simulink model "SIMULINK_PID_Tracking_R18b"  (R2018b)
settings: Solver=FixedStepAuto  StartTime=0.0  StopTime=sim_end_time  FixedStep=fixed_step_size  RelTol=1e-3
undefined symbols (not defined in the file): a, act_end, b, battery_threshold, bb, draw_gif, droneyeeUAV2_NUM, droneyeeUAV3_NUM, droneyeeUAV4_NUM, droneyeeUAV5_NUM, fixed_step_size, k, KD_x, KD_y, kd_z, KDD_x, KDD_y, KI_x, KI_y, ki_z, KII_x, KII_y, KP_x, KP_y, kp_z, KPP_x, KPP_y, lmt, omega, R, sim_end_time, uav10num, uav1num, uav2num, uav3num, uav4num, uav5num, uav6num, uav7num, uav8num, uav9num, UAV_NUM, Vel_Switch_1, Vel_Switch_10, Vel_Switch_11, Vel_Switch_12, Vel_Switch_13, Vel_Switch_14, Vel_Switch_15, Vel_Switch_16, Vel_Switch_17, Vel_Switch_18, Vel_Switch_19, Vel_Switch_2, Vel_Switch_20, Vel_Switch_3, Vel_Switch_4, Vel_Switch_5, Vel_Switch_6, Vel_Switch_7 ... (+12)
libraries: simulink x120, aerolibanimutils x1
(part 10 of 10)

== matlab function SIMULINK_PID_Tracking_R18b/防碰撞2/MATLAB Function ==
  settings: updateMethod=DISCRETE
  data: u1 input; xd output; u2 input; yd output; zd output; u3 input; u4 input; u5 input; flag input
function [xd,yd,zd] = fcn(u1,u2,u3,u4,u5,flag)
persistent xdd ydd zdd xtt ytt ztt;
k=u4;
totnum =10;
safedist =u3;%安全距离的平方
bang=u5;
xdd=zeros(totnum,1);
ydd=zeros(totnum,1);
zdd=zeros(totnum,1);
xt=zeros(totnum,1);
yt=zeros(totnum,1);
zt=zeros(totnum,1);
vx=xt;
vy=yt;
vz=zt;
xd=xt;
yd=yt;
zd=zt;
for i =1:1:totnum
    xt(i)=u2(12*(i-1)+1);
    yt(i)=u2(12*(i-1)+2);
    zt(i)=u2(12*(i-1)+3);
    xd(i)=u1(6*(i-1)+1);
    yd(i)=u1(6*(i-1)+2);
    zd(i)=u1(6*(i-1)+3);
    vx(i)=u2(12*(i-1)+10);
    vy(i)=u2(12*(i-1)+11);
    vz(i)=u2(12*(i-1)+12);
end
if flag==1
if isempty(xt)
    xtt = xt;
    ytt = yt;
    ztt = zt;
end
for i =1:1:(totnum-1)
    if xt(i)==0&&yt(i)==0&&zt(i)==0
        break
    end
    for j=(i+1):1:totnum
        if xt(j)==0&&yt(j)==0&&zt(j)==0
        break
        end
        dist=((xt(i)-xt(j))^2+(yt(i)-yt(j))^2+(zt(i)-zt(j))^2);
        sqrt_dist=sqrt((xt(i)-xt(j))^2+(yt(i)-yt(j))^2);
    if (dist>0)&&(sqrt(dist)<=bang)
%         xd(i)=xt(i);
%         yd(i)=yt(i);
%         zd(i)=0; %zt(i);
%         xd(j)=xt(j);
%         yd(j)=yt(j);
%         zd(j)=zt(j);        
%         xd(i)=xd(i)+k*(xt(i)-xt(j))*(safedist-dist);
%         yd(i)=yd(i)+k*(yt(i)-yt(j))*(safedist-dist);
        xdd(i)=xdd(i)+k*(xt(i)-xt(j))*(safedist-dist);
        ydd(i)=ydd(i)+k*(yt(i)-yt(j))*(safedist-dist);
%         zd(i)=zd(i)+k*(zt(i)-zt(j))*(safedist-dist);
%         xd(j)=xd(j)-k*(xt(i)-xt(j))*(safedist-dist);
%         yd(j)=yd(j)-k*(yt(i)-yt(j))*(safedist-dist);
        xdd(j)=xdd(j)-k*(xt(i)-xt(j))*(safedist-dist);
        ydd(j)=ydd(j)-k*(yt(i)-yt(j))*(safedist-dist);
%         zd(j)=zd(j)-k*(zt(i)-zt(j))*(safedist-dist);
     elseif (sqrt(dist)<safedist)&&(((vx(i)-vx(j))*(xt(i)-xt(j))+...
             (vy(i)-vy(j))*(yt(i)-yt(j)))<0)
%         dist=dist-bang;
%         xd(i)=xd(i)+k*(yt(i)-yt(j))*(safedist-dist);
%         yd(i)=yd(i)+k*(xt(j)-xt(i))*(safedist-dist);
        xdd(i)=xdd(i)+k*(yt(i)-yt(j))*(safedist-sqrt_dist)/sqrt_dist/sqrt_dist;
        ydd(i)=ydd(i)+k*(xt(j)-xt(i))*(safedist-sqrt_dist)/sqrt_dist/sqrt_dist;
%         zd(i)=zd(i)+k*(zt(i)-zt(j))*(safedist-dist);
%         xd(j)=xd(j)-k*(yt(i)-yt(j))*(safedist-dist);
%         yd(j)=yd(j)-k*(xt(j)-xt(i))*(safedist-dist);
        xdd(j)=xdd(j)-k*(yt(i)-yt(j))*(safedist-sqrt_dist)/sqrt_dist/sqrt_dist;
        ydd(j)=ydd(j)-k*(xt(j)-xt(i))*(safedist-sqrt_dist)/sqrt_dist/sqrt_dist;
%         zd(j)=zd(j)-k*(zt(i)-zt(j))*(safedist-dist);
        
    end
    end
end
xd=xd+xdd;
yd=yd+ydd;
% zd=zdd;
end

== matlab function SIMULINK_PID_Tracking_R18b/control system_UAV/Baseline Controller3/MATLAB Function ==
  data: u input; y output; a input
function y = fcn(u,a)
y = satgd(u,a);

== matlab function SIMULINK_PID_Tracking_R18b/CMD_car1/CMD6/Subsystem/MATLAB Function ==
  settings: updateMethod=DISCRETE
  data: timestamp input; uavnum input; x_ output; y_ output; z_ output; switch_flag input; stas input; trj_flag input; form_flag input; avo_flag input
function [x_, y_, z_] = fcn(timestamp, uavnum,switch_flag,stas,trj_flag,form_flag,avo_flag)

[x_,y_,z_]=trjcar(timestamp,uavnum,switch_flag,stas,trj_flag,form_flag,avo_flag);

== matlab function SIMULINK_PID_Tracking_R18b/control system_UAV/Baseline Controller4/MATLAB Function ==
  data: u input; y output; a input
function y = fcn(u,a)
y = satgd(u,a);

== matlab function SIMULINK_PID_Tracking_R18b/CMD_car1/CMD7/MATLAB Function1 ==
  settings: updateMethod=DISCRETE
  data: x_d input; y_d input; z_d input; timestamp input; x input; y input; z input; battery_status input; sim_time_end input; x_d_ output; battery_threshold input; z_d_for_land input; y_d_ output; z_d_ output; UAV_NUM input
function [x_d_, y_d_, z_d_] = fcn(x_d, y_d, z_d, timestamp, x,y,z,battery_status, sim_time_end,battery_threshold, z_d_for_land, UAV_NUM)
persistent s_x s_y s_z ready_land
if isempty(s_x)
    s_x = x;
end
if isempty(s_y)
    s_y = y;
end
if isempty(s_z)
    s_z = z;
end
if isempty(ready_land)
    ready_land = false;
end
    
battery_low = false;
for i = 1:UAV_NUM
    if battery_status(i) < battery_threshold
        battery_low = true;
        break;
    end
end
if sim_time_end - timestamp < 1
    tello_stop = true;
else
    tello_stop = false;
end
if battery_low || tello_stop
    if ~ready_land
        ready_land = true;
    end
    z_d_ = z_d_for_land;
    x_d_ = s_x;
    y_d_ = s_y;
else
   ready_land = false;
   s_x = x;
   s_y = y;
   x_d_ = x_d;
   y_d_ = y_d;
   z_d_ = z_d;
end

== matlab function SIMULINK_PID_Tracking_R18b/CMD_UAV/CMD6/Subsystem/MATLAB Function ==
  settings: updateMethod=DISCRETE
  data: timestamp input; uavnum input; x_ output; y_ output; z_ output; switch_flag input; stas input; trj_flag input; form_flag input; avo_flag input
function [x_, y_, z_] = fcn(timestamp, uavnum,switch_flag,stas,trj_flag,form_flag,avo_flag)

[x_,y_,z_]=trjuav(timestamp,uavnum,switch_flag,stas,trj_flag,form_flag,avo_flag);

== matlab function SIMULINK_PID_Tracking_R18b/CMD_UAV/CMD7/MATLAB Function1 ==
  settings: updateMethod=DISCRETE
  data: x_d input; y_d input; z_d input; timestamp input; x input; y input; z input; battery_status input; sim_time_end input; x_d_ output; battery_threshold input; z_d_for_land input; y_d_ output; z_d_ output; UAV_NUM input
function [x_d_, y_d_, z_d_] = fcn(x_d, y_d, z_d, timestamp, x,y,z,battery_status, sim_time_end,battery_threshold, z_d_for_land, UAV_NUM)
persistent s_x s_y s_z ready_land
if isempty(s_x)
    s_x = x;
end
if isempty(s_y)
    s_y = y;
end
if isempty(s_z)
    s_z = z;
end
if isempty(ready_land)
    ready_land = false;
end
    
battery_low = false;
for i = 1:UAV_NUM
    if battery_status(i) < battery_threshold
        battery_low = true;
        break;
    end
end
if sim_time_end - timestamp < 1
    tello_stop = true;
else
    tello_stop = false;
end
if battery_low || tello_stop
    if ~ready_land
        ready_land = true;
    end
    z_d_ = z_d_for_land;
    x_d_ = s_x;
    y_d_ = s_y;
else
   ready_land = false;
   s_x = x;
   s_y = y;
   x_d_ = x_d;
   y_d_ = y_d;
   z_d_ = z_d;
end

== matlab function SIMULINK_PID_Tracking_R18b/CMD_UAV/CMD7/Subsystem/MATLAB Function ==
  settings: updateMethod=DISCRETE
  data: timestamp input; uavnum input; x_ output; y_ output; z_ output; switch_flag input; stas input; trj_flag input; form_flag input; avo_flag input
function [x_, y_, z_] = fcn(timestamp, uavnum,switch_flag,stas,trj_flag,form_flag,avo_flag)

[x_,y_,z_]=trjuav(timestamp,uavnum,switch_flag,stas,trj_flag,form_flag,avo_flag);

== matlab function SIMULINK_PID_Tracking_R18b/CMD_UAV/CMD8/MATLAB Function1 ==
  settings: updateMethod=DISCRETE
  data: x_d input; y_d input; z_d input; timestamp input; x input; y input; z input; battery_status input; sim_time_end input; x_d_ output; battery_threshold input; z_d_for_land input; y_d_ output; z_d_ output; UAV_NUM input
function [x_d_, y_d_, z_d_] = fcn(x_d, y_d, z_d, timestamp, x,y,z,battery_status, sim_time_end,battery_threshold, z_d_for_land, UAV_NUM)
persistent s_x s_y s_z ready_land
if isempty(s_x)
    s_x = x;
end
if isempty(s_y)
    s_y = y;
end
if isempty(s_z)
    s_z = z;
end
if isempty(ready_land)
    ready_land = false;
end
    
battery_low = false;
for i = 1:UAV_NUM
    if battery_status(i) < battery_threshold
        battery_low = true;
        break;
    end
end
if sim_time_end - timestamp < 1
    tello_stop = true;
else
    tello_stop = false;
end
if battery_low || tello_stop
    if ~ready_land
        ready_land = true;
    end
    z_d_ = z_d_for_land;
    x_d_ = s_x;
    y_d_ = s_y;
else
   ready_land = false;
   s_x = x;
   s_y = y;
   x_d_ = x_d;
   y_d_ = y_d;
   z_d_ = z_d;
end

== matlab function SIMULINK_PID_Tracking_R18b/CMD_UAV/CMD8/Subsystem/MATLAB Function ==
  settings: updateMethod=DISCRETE
  data: timestamp input; uavnum input; x_ output; y_ output; z_ output; switch_flag input; stas input; trj_flag input; form_flag input; avo_flag input
function [x_, y_, z_] = fcn(timestamp, uavnum,switch_flag,stas,trj_flag,form_flag,avo_flag)

[x_,y_,z_]=trjuav(timestamp,uavnum,switch_flag,stas,trj_flag,form_flag,avo_flag);

== matlab function SIMULINK_PID_Tracking_R18b/CMD_UAV/CMD10/MATLAB Function1 ==
  settings: updateMethod=DISCRETE
  data: x_d input; y_d input; z_d input; timestamp input; x input; y input; z input; battery_status input; sim_time_end input; x_d_ output; battery_threshold input; z_d_for_land input; y_d_ output; z_d_ output; UAV_NUM input
function [x_d_, y_d_, z_d_] = fcn(x_d, y_d, z_d, timestamp, x,y,z,battery_status, sim_time_end,battery_threshold, z_d_for_land, UAV_NUM)
persistent s_x s_y s_z ready_land
if isempty(s_x)
    s_x = x;
end
if isempty(s_y)
    s_y = y;
end
if isempty(s_z)
    s_z = z;
end
if isempty(ready_land)
    ready_land = false;
end
    
battery_low = false;
for i = 1:UAV_NUM
    if battery_status(i) < battery_threshold
        battery_low = true;
        break;
    end
end
if sim_time_end - timestamp < 1
    tello_stop = true;
else
    tello_stop = false;
end
if battery_low || tello_stop
    if ~ready_land
        ready_land = true;
    end
    z_d_ = z_d_for_land;
    x_d_ = s_x;
    y_d_ = s_y;
else
   ready_land = false;
   s_x = x;
   s_y = y;
   x_d_ = x_d;
   y_d_ = y_d;
   z_d_ = z_d;
end

== matlab function SIMULINK_PID_Tracking_R18b/CMD_UAV/CMD10/Subsystem/MATLAB Function ==
  settings: updateMethod=DISCRETE
  data: timestamp input; uavnum input; x_ output; y_ output; z_ output; switch_flag input; stas input; trj_flag input; form_flag input; avo_flag input
function [x_, y_, z_] = fcn(timestamp, uavnum,switch_flag,stas,trj_flag,form_flag,avo_flag)

[x_,y_,z_]=trjuav(timestamp,uavnum,switch_flag,stas,trj_flag,form_flag,avo_flag);

== matlab function SIMULINK_PID_Tracking_R18b/CMD_UAV/CMD9/MATLAB Function1 ==
  settings: updateMethod=DISCRETE
  data: x_d input; y_d input; z_d input; timestamp input; x input; y input; z input; battery_status input; sim_time_end input; x_d_ output; battery_threshold input; z_d_for_land input; y_d_ output; z_d_ output; UAV_NUM input
function [x_d_, y_d_, z_d_] = fcn(x_d, y_d, z_d, timestamp, x,y,z,battery_status, sim_time_end,battery_threshold, z_d_for_land, UAV_NUM)
persistent s_x s_y s_z ready_land
if isempty(s_x)
    s_x = x;
end
if isempty(s_y)
    s_y = y;
end
if isempty(s_z)
    s_z = z;
end
if isempty(ready_land)
    ready_land = false;
end
    
battery_low = false;
for i = 1:UAV_NUM
    if battery_status(i) < battery_threshold
        battery_low = true;
        break;
    end
end
if sim_time_end - timestamp < 1
    tello_stop = true;
else
    tello_stop = false;
end
if battery_low || tello_stop
    if ~ready_land
        ready_land = true;
    end
    z_d_ = z_d_for_land;
    x_d_ = s_x;
    y_d_ = s_y;
else
   ready_land = false;
   s_x = x;
   s_y = y;
   x_d_ = x_d;
   y_d_ = y_d;
   z_d_ = z_d;
end

== matlab function SIMULINK_PID_Tracking_R18b/CMD_UAV/CMD9/Subsystem/MATLAB Function ==
  settings: updateMethod=DISCRETE
  data: timestamp input; uavnum input; x_ output; y_ output; z_ output; switch_flag input; stas input; trj_flag input; form_flag input; avo_flag input
function [x_, y_, z_] = fcn(timestamp, uavnum,switch_flag,stas,trj_flag,form_flag,avo_flag)

[x_,y_,z_]=trjuav(timestamp,uavnum,switch_flag,stas,trj_flag,form_flag,avo_flag);

== matlab function SIMULINK_PID_Tracking_R18b/CMD_car1/CMD7/Subsystem/MATLAB Function ==
  settings: updateMethod=DISCRETE
  data: timestamp input; uavnum input; x_ output; y_ output; z_ output; switch_flag input; stas input; trj_flag input; form_flag input; avo_flag input
function [x_, y_, z_] = fcn(timestamp, uavnum,switch_flag,stas,trj_flag,form_flag,avo_flag)

[x_,y_,z_]=trjcar(timestamp,uavnum,switch_flag,stas,trj_flag,form_flag,avo_flag);

== matlab function SIMULINK_PID_Tracking_R18b/CMD_car1/CMD8/MATLAB Function1 ==
  settings: updateMethod=DISCRETE
  data: x_d input; y_d input; z_d input; timestamp input; x input; y input; z input; battery_status input; sim_time_end input; x_d_ output; battery_threshold input; z_d_for_land input; y_d_ output; z_d_ output; UAV_NUM input
function [x_d_, y_d_, z_d_] = fcn(x_d, y_d, z_d, timestamp, x,y,z,battery_status, sim_time_end,battery_threshold, z_d_for_land, UAV_NUM)
persistent s_x s_y s_z ready_land
if isempty(s_x)
    s_x = x;
end
if isempty(s_y)
    s_y = y;
end
if isempty(s_z)
    s_z = z;
end
if isempty(ready_land)
    ready_land = false;
end
    
battery_low = false;
for i = 1:UAV_NUM
    if battery_status(i) < battery_threshold
        battery_low = true;
        break;
    end
end
if sim_time_end - timestamp < 1
    tello_stop = true;
else
    tello_stop = false;
end
if battery_low || tello_stop
    if ~ready_land
        ready_land = true;
    end
    z_d_ = z_d_for_land;
    x_d_ = s_x;
    y_d_ = s_y;
else
   ready_land = false;
   s_x = x;
   s_y = y;
   x_d_ = x_d;
   y_d_ = y_d;
   z_d_ = z_d;
end

== matlab function SIMULINK_PID_Tracking_R18b/CMD_car1/CMD8/Subsystem/MATLAB Function ==
  settings: updateMethod=DISCRETE
  data: timestamp input; uavnum input; x_ output; y_ output; z_ output; switch_flag input; stas input; trj_flag input; form_flag input; avo_flag input
function [x_, y_, z_] = fcn(timestamp, uavnum,switch_flag,stas,trj_flag,form_flag,avo_flag)

[x_,y_,z_]=trjcar(timestamp,uavnum,switch_flag,stas,trj_flag,form_flag,avo_flag);

== matlab function SIMULINK_PID_Tracking_R18b/CMD_car1/CMD9/MATLAB Function1 ==
  settings: updateMethod=DISCRETE
  data: x_d input; y_d input; z_d input; timestamp input; x input; y input; z input; battery_status input; sim_time_end input; x_d_ output; battery_threshold input; z_d_for_land input; y_d_ output; z_d_ output; UAV_NUM input
function [x_d_, y_d_, z_d_] = fcn(x_d, y_d, z_d, timestamp, x,y,z,battery_status, sim_time_end,battery_threshold, z_d_for_land, UAV_NUM)
persistent s_x s_y s_z ready_land
if isempty(s_x)
    s_x = x;
end
if isempty(s_y)
    s_y = y;
end
if isempty(s_z)
    s_z = z;
end
if isempty(ready_land)
    ready_land = false;
end
    
battery_low = false;
for i = 1:UAV_NUM
    if battery_status(i) < battery_threshold
        battery_low = true;
        break;
    end
end
if sim_time_end - timestamp < 1
    tello_stop = true;
else
    tello_stop = false;
end
if battery_low || tello_stop
    if ~ready_land
        ready_land = true;
    end
    z_d_ = z_d_for_land;
    x_d_ = s_x;
    y_d_ = s_y;
else
   ready_land = false;
   s_x = x;
   s_y = y;
   x_d_ = x_d;
   y_d_ = y_d;
   z_d_ = z_d;
end

== matlab function SIMULINK_PID_Tracking_R18b/CMD_car1/CMD9/Subsystem/MATLAB Function ==
  settings: updateMethod=DISCRETE
  data: timestamp input; uavnum input; x_ output; y_ output; z_ output; switch_flag input; stas input; trj_flag input; form_flag input; avo_flag input
function [x_, y_, z_] = fcn(timestamp, uavnum,switch_flag,stas,trj_flag,form_flag,avo_flag)

[x_,y_,z_]=trjcar(timestamp,uavnum,switch_flag,stas,trj_flag,form_flag,avo_flag);

== matlab function SIMULINK_PID_Tracking_R18b/control system_car1/Baseline Controller1/MATLAB Function ==
  data: u input; y output; a input
function y = fcn(u,a)
y = satgd(u,a);

== matlab function SIMULINK_PID_Tracking_R18b/control system_car1/Baseline Controller2/MATLAB Function ==
  data: u input; y output; a input
function y = fcn(u,a)
y = satgd(u,a);

== matlab function SIMULINK_PID_Tracking_R18b/control system_car1/Baseline Controller3/MATLAB Function ==
  data: u input; y output; a input
function y = fcn(u,a)
y = satgd(u,a);

== matlab function SIMULINK_PID_Tracking_R18b/control system_car1/Baseline Controller4/MATLAB Function ==
  data: u input; y output; a input
function y = fcn(u,a)
y = satgd(u,a);

== matlab function SIMULINK_PID_Tracking_R18b/control system_car1/Baseline Controller5/MATLAB Function ==
  data: u input; y output; a input
function y = fcn(u,a)
y = satgd(u,a);

== matlab function SIMULINK_PID_Tracking_R18b/control system_car1/MATLAB Function ==
  data: u input; y output
function y = fcn(u)
plot(u(1),u(2),"*");
hold on;
y = u;

== matlab function SIMULINK_PID_Tracking_R18b/control system_car1/Baseline Controller6/MATLAB Function ==
  data: u input; y output; a input
function y = fcn(u,a)
y = satgd(u,a);

== matlab function SIMULINK_PID_Tracking_R18b/control system_car1/Baseline Controller7/MATLAB Function ==
  data: u input; y output; a input
function y = fcn(u,a)
y = satgd(u,a);

== matlab function SIMULINK_PID_Tracking_R18b/control system_car1/Baseline Controller8/MATLAB Function ==
  data: u input; y output; a input
function y = fcn(u,a)
y = satgd(u,a);

== matlab function SIMULINK_PID_Tracking_R18b/control system_car1/Baseline Controller9/MATLAB Function ==
  data: u input; y output; a input
function y = fcn(u,a)
y = satgd(u,a);

== matlab function SIMULINK_PID_Tracking_R18b/防碰撞1/MATLAB Function1 ==
  settings: updateMethod=DISCRETE
  data: u1 input; xd output; u2 input; yd output; zd output; u3 input; u4 input; u5 input; flag input
function [xd,yd,zd] = fcn(u1,u2,u3,u4,u5,flag)

persistent xdd ydd zdd xtt ytt ztt;
k=u4;
totnum =10;
safedist =u3;%安全距离
bang=u5;
xdd=zeros(totnum,1);
ydd=zeros(totnum,1);
zdd=zeros(totnum,1);
xt=zeros(totnum,1);
yt=zeros(totnum,1);
zt=zeros(totnum,1);
vx=xt;
vy=yt;
vz=zt;
xd=xt;
yd=yt;
zd=zt;

for i =1:1:totnum
    xt(i)=u2(12*(i-1)+1);
    yt(i)=u2(12*(i-1)+2);
    zt(i)=u2(12*(i-1)+3);
    vx(i)=u2(12*(i-1)+10);
    vy(i)=u2(12*(i-1)+11);
    vz(i)=u2(12*(i-1)+12);
    xd(i)=u1(4*(i-1)+1);
    yd(i)=u1(4*(i-1)+2);
    zd(i)=u1(4*(i-1)+3);
end
if flag==1
    if isempty(xtt)
        xtt = xt;
        ytt = yt;
        ztt = zt;
    end
    for i =1:1:(totnum-1)
        if (xt(i)==0)&&(yt(i)==0)&&(zt(i)==0)
            continue
        end
        for j=(i+1):1:totnum
            if xt(j)==0 && yt(j)==0 && zt(j)==0
                continue
            end
            dist=(xt(i)-xt(j))^2+(yt(i)-yt(j))^2+(zt(i)-zt(j))^2;
            sqrt_dist=sqrt((xt(i)-xt(j))^2+(yt(i)-yt(j))^2);
            if (dist>0)&&(sqrt(dist)<bang)
                %         xdd(i)=xtt(i);
                %         ydd(i)=ytt(i);
                %         zdd(i)=ztt(i);
                %         xdd(j)=xtt(j);
                %         ydd(j)=ytt(j);
                %         zdd(j)=ztt(j);
                xdd(i)=k*(xt(i)-xt(j))*(safedist-sqrt_dist)/dist;
                ydd(i)=k*(yt(i)-yt(j))*(safedist-sqrt_dist)/dist;
                %         zdd(i)=zt(i)+k*(zt(i)-zt(j))*(safedist-sqrt_dist)/sqrt_dist;
                xdd(j)=-k*(xt(i)-xt(j))*(safedist-sqrt_dist)/dist;
                ydd(j)=-k*(yt(i)-yt(j))*(safedist-sqrt_dist)/dist;
                %         zdd(j)=zt(j)-k*(zt(i)-zt(j))*(safedist-dist)/sqrt_dist;
                
            elseif (sqrt(dist)<safedist)&&(((vx(i)-vx(j))*(xt(i)-xt(j))+...
                    (vy(i)-vy(j))*(yt(i)-yt(j)))<0)
                %         xdd(i)=(xdd(i)+xt(i)+k*(yt(i)-yt(j))*(safedist-sqrt_dist)/dist)/(k*(safedist-sqrt_dist)/dist+1);
                %         ydd(i)=(ydd(i)+yt(i)+k*(xt(j)-xt(i))*(safedist-sqrt_dist)/dist)/(k*(safedist-sqrt_dist)/dist+1);
                %         zdd(i)=zdd(i)+k*(zt(i)-zt(j))*(safedist-sqrt_dist)/sqrt_dist;
                %         xdd(j)=(xdd(j)+xt(j)-k*(yt(i)-yt(j))*(safedist-sqrt_dist)/dist)/(k*(safedist-sqrt_dist)/dist+1);
                %         ydd(j)=(ydd(j)+yt(j)-k*(xt(j)-xt(i))*(safedist-sqrt_dist)/dist)/(k*(safedist-sqrt_dist)/dist+1);
                %         zdd(j)=zdd(j)-k*(zt(i)-zt(j))*(safedist-sqrt_dist)/sqrt_dist;
                %
                %         xdd(i)=(xt(i)+k*(yt(i)-yt(j))*(safedist-sqrt_dist)/dist)/(k*(safedist-sqrt_dist)/dist+1);
                %         ydd(i)=(yt(i)+k*(xt(j)-xt(i))*(safedist-sqrt_dist)/dist)/(k*(safedist-sqrt_dist)/dist+1);
                %         zdd(i)=zdd(i)+k*(zt(i)-zt(j))*(safedist-sqrt_dist)/sqrt_dist;
                %         xdd(j)=(xt(j)-k*(yt(i)-yt(j))*(safedist-sqrt_dist)/dist)/(k*(safedist-sqrt_dist)/dist+1);
                %         ydd(j)=(yt(j)-k*(xt(j)-xt(i))*(safedist-sqrt_dist)/dist)/(k*(safedist-sqrt_dist)/dist+1);
                %         zdd(j)=zdd(j)-k*(zt(i)-zt(j))*(safedist-sqrt_dist)/sqrt_dist;
                
                xdd(i)=(xdd(i)+k*(yt(i)-yt(j))*(safedist-sqrt_dist)/dist);
                ydd(i)=(ydd(i)+k*(xt(j)-xt(i))*(safedist-sqrt_dist)/dist);
                %         zdd(i)=zdd(i)+k*(zt(i)-zt(j))*(safedist-sqrt_dist)/sqrt_dist;
                xdd(j)=(xdd(j)-k*(yt(i)-yt(j))*(safedist-sqrt_dist)/dist);
                ydd(j)=(ydd(j)-k*(xt(j)-xt(i))*(safedist-sqrt_dist)/dist);
                %         zdd(j)=zdd(j)-k*(zt(i)-zt(j))*(safedist-sqrt_dist)/sqrt_dist;
                
            end
        end
        
    end
    
    for m =1:1:totnum
        if (xdd(m) ~= 0)||(ydd(m)~= 0)
            xd(m)=xdd(m)+xt(m);
            yd(m)=ydd(m)+yt(m);
        end
    end
    % zd=zdd;
    
    
end
end

== matlab function SIMULINK_PID_Tracking_R18b/control system_car1/Baseline Controller10/MATLAB Function ==
  data: u input; y output; a input
function y = fcn(u,a)
y = satgd(u,a);
